simulink model "cordic_cycle"  (R2017a)
settings: Solver=FixedStepDiscrete  StartTime=0.0  StopTime=100  RelTol=1e-3  EnableMultiTasking=on
InitFcn:
  | %% DSPBuilder Start
  | alt_dspbuilder_update_model(bdroot)
  | %% DSPBuilder End
StartFcn:
  | %% DSPBuilder Start
  | alt_dspbuilder_hdlimport_prepare_for_simulation(bdroot)
  | %% DSPBuilder End
undefined symbols (not defined in the file or in its folder): AdvDSPBChannelOutDisplay, dpoly, dspba, dspba_ChannelInVis, dspba_ChannelOutVis, dspba_internal_get_channel_ports, evalAionMaskParam, latency, primtype, value
libraries: DSPBAPrim x101, DSPBAControl x12, DSPBABase x3, simulink x3
settings Model: Creator=lkong  LastModifiedBy=hatikvah
settings DataIOCC: LimitDataPoints=on  SaveFormat=Array  SignalLoggingSaveFormat=ModelDataLogs
settings OptimizationCC: ExpressionDepthLimit=2147483647  InitFltsAndDblsToZero=on  LifeSpan=inf
settings DebuggingCC: SaveWithParameterizedLinksMsg=none  UnderspecifiedInitializationDetection=Classic  MergeDetectMultiDrivingBlocksExec=none  SignalResolutionControl=TryResolveAllWithWarning  SolverPrmCheckMsg=warning  MultiTaskDSMMsg=warning  MultiTaskCondExecSysMsg=none  FcnCallInpInsideContextMsg=warning  StateNameClashWarn=warning  SFUnexpectedBacktrackingDiag=warning  SFNoUnconditionalDefaultTransitionDiag=warning  SFExecutionAtInitializationDiag=none
settings HardwareCC: ProdBitPerPointer=32  ProdBitPerSizeT=32  ProdBitPerPtrDiffT=32  ProdLargestAtomicFloat=None  ProdIntDivRoundTo=Undefined  ProdEndianess=Unspecified  ProdWordSize=32  ProdHWDeviceType=32-bit Generic
settings ModelReferenceCC: PropagateSignalLabelsOutOfModel=off
settings GRTTargetCC: TargetFcnLib=ansi_tfl_tmw.mat  TargetLangStandard=C89/C90 (ANSI)  GeneratePreprocessorConditionals=Disable all  CombineOutputUpdateFcns=off  GRTInterface=on
settings ConfigComp: CovMetricSettings=dw  CovHtmlReporting=on  CovSaveCumulativeToWorkspaceVar=on  CovSaveSingleToWorkspaceVar=on  CovExternalEMLEnable=off

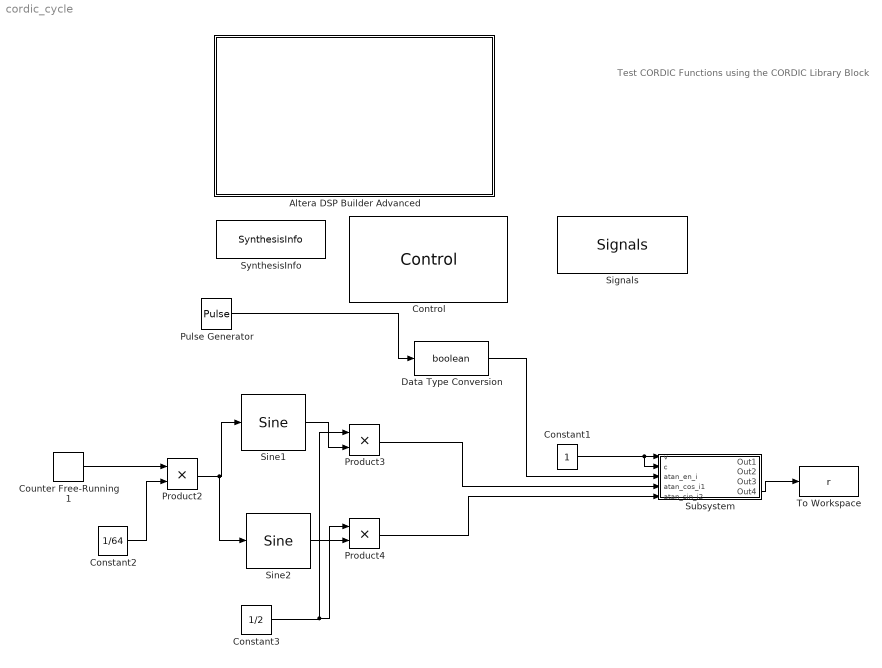
== system cordic_cycle ==
  note: Test CORDIC Functions
      | using the CORDIC Library Block
  Altera DSP Builder Advanced : Subsystem  mask(DSP Builder Advanced Blockset Ignored Block){}
      settings: OpenFcn=web('http://www.altera.com', '-new');
      mask Display: image(imread('intellogo.tif'));
  Constant1 : Constant  OutDataTypeStr=boolean  LockScale=on
  Constant2 : Constant  Value=1/64  OutDataTypeStr=double  LockScale=on
  Constant3 : Constant  Value=1/2  OutDataTypeStr=fixdt(1,32,31)  LockScale=on
  Control : DSPBABase/Control  generate=on  language=VHDL  destination=../rtl  destination_gui=../rtl  make_full_path=off  path_is_relative=on  autotestbench=on  signaldepth=3  coveragetestbench=off  logs=off  spacewidth=2  spacenum=1  addrwidth=10  datawidth=16  dataendian=Big Endian  hierarchicalnames=on  ramThresholdBits=20  distRamThresholdBits=-1  mlabThresholdBits=-1  hardMultiplierThresholdLuts=-1  version=20090407  errorOnChanMismatch=1  errorOnGPIOMismatch=0  importModelsimResults=0  cycleAccurate=off  reinterpretCastMult=off  paramFile=cordic_cycle_params.xml
  Counter Free-Running1 : simulink/Sources/Counter Free-Running  NumBits=10  tsamp=-1
  Data Type Conversion : DataTypeConversion  OutDataTypeStr=boolean
  Product2 : Product
  Product3 : Product  OutDataTypeStr=Inherit: Same as first input  LockScale=on
  Product4 : Product  OutDataTypeStr=Inherit: Same as first input  LockScale=on
  Pulse Generator : DiscretePulseGenerator  PulseType=Time based  Period=10  PulseWidth=2
  Signals : DSPBABase/Signals  clk=clk  freq=50  margin=0  rst=areset  rstactive=High  bus=bus  enbusclock=off  busfreq=50  bussync=off  version=20090407
  Sine1 : simulink/Lookup Tables/Sine  Formula=cos(2*pi*u)  NumDataPoints=(2^5)+1  OutputWordLength=32  InternalRulePriority=Speed
      settings: SourceProductName=Simulink
  Sine2 : simulink/Lookup Tables/Sine  Formula=sin(2*pi*u)  NumDataPoints=(2^5)+1  OutputWordLength=32  InternalRulePriority=Speed
      settings: SourceProductName=Simulink
  Subsystem : Subsystem
  SynthesisInfo : DSPBAPrim/SynthesisInfo  primtype=synthinfo  nInputs=0  nOutputs=0  omode=Inherit via internal rule  otype=sfix(16)  scale=2^-15  rndmethod=Truncate  factor=1  satmethod=Symmetric  shift_vec=[0 1 2 -1]  value=99  inPortNames=[' '; ' ';]  outPortNames=[' ']  dspbaimage=dspba_prim_ctrl.jpg  text=fprintf('Style=%s', style);  style=Scheduled  visibilities=2^17+2^18+2^19+2^20  constraintInUse=off  constraintRelation=>  constraintLimit=2  bitAccurate=off  version=20150220
  To Workspace : ToWorkspace  VariableName=r  SaveFormat=Timeseries  SampleTime=-1
  wires:
  Constant2/1 -> Product2/2
  Product2/1 -> Sine2/1, Sine1/1
  Product3/1 -> Subsystem/4(atan_cos_i1)
  Product4/1 -> Subsystem/5(atan_sin_i2)
  Pulse Generator/1 -> Data Type Conversion/1
  Sine1/1 -> Product3/2
  Sine2/1 -> Product4/2
  Constant3/1 -> Product4/1, Product3/1
  Counter Free-Running1/1 -> Product2/1
  Data Type Conversion/1 -> Subsystem/3(atan_en_i)
  Constant1/1 -> Subsystem/2(c), Subsystem/1(v)
  Subsystem/4(Out4) -> To Workspace/1

== system cordic_cycle/Altera DSP Builder Advanced ==

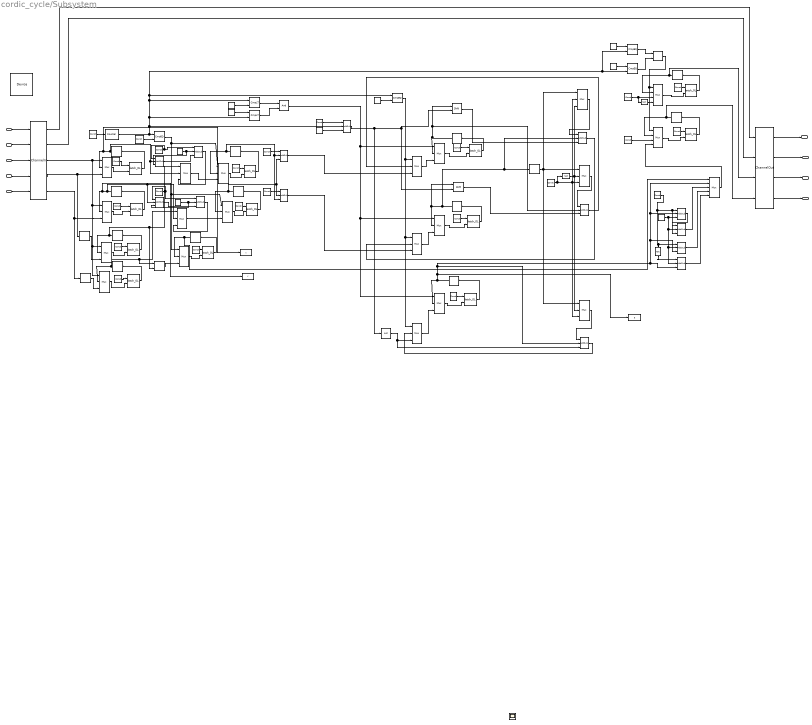
== system cordic_cycle/Subsystem ==
  v : Inport  OutDataTypeStr=boolean
  c : Inport  Port=2
  atan_en_i : Inport  Port=3
  atan_cos_i1 : Inport  Port=4
  atan_sin_i2 : Inport  Port=5
  AddSub{,1..13} (14 alike) : DSPBAPrim/AddSub  primtype=addsub  nInputs=3  nOutputs=1  omode=Inherit via internal rule  otype=sfix(16)  scale=2^-15  rndmethod=Unbiased  factor=1  satmethod=Symmetric  shift_vec=[0 1 2 -1]  value=0  inPortNames="['add'; 'x  '; 'y  ']"  outPortNames=[' ']  dspbaimage=dspba_prim.jpg  text=fprintf('add\nsub');  style=Optimised  visibilities=8+2^17+2^18  floatRounding=correct  advOptions=[]  version=20130110
  And : DSPBAPrim/And  primtype=and  nInputs=2  nOutputs=1  omode=Inherit via internal rule  otype=sfix(16)  scale=2^-15  rndmethod=Unbiased  factor=1  satmethod=Symmetric  shift_vec=[0 1 2 -1]  value=0  inPortNames=[' '; ' '; ' '; ' '; ' '; ' '; ' '; ' '; ' '; ' '; ' '; ' '; ' '; ' '; ' '; ' '; ]  outPortNames=[' ']  dspbaimage=dspba_prim.jpg  text=fprintf('&');  style=Optimised  visibilities=8+2  version=20090407
  BitCombine : DSPBAPrim/BitCombine  primtype=bitcombine  nInputs=2  nOutputs=1  omode=Inherit via internal rule  otype=sfix(16)  scale=2^-15  rndmethod=Unbiased  factor=1  satmethod=Symmetric  shift_vec=[0 1 2 -1]  value=0  inPortNames=['l'; 'h';]  outPortNames=[' ']  dspbaimage=dspba_prim.jpg  text=fprintf('[h,l]');  style=Optimised  visibilities=8+2  version=20090407
  BitCombine1 : DSPBAPrim/BitCombine  primtype=bitcombine  nInputs=2  nOutputs=1  omode=Inherit via internal rule  otype=sfix(16)  scale=2^-15  rndmethod=Unbiased  factor=1  satmethod=Symmetric  shift_vec=[0 1 2 -1]  value=0  inPortNames=['l'; 'h';]  outPortNames=[' ']  dspbaimage=dspba_prim.jpg  text=fprintf('[h,l]');  style=Optimised  visibilities=8+2  version=20090407
  ChannelIn : DSPBAPrim/ChannelIn  primtype=channelin  nInputs=dspba_internal_get_channel_ports(gcb)  nOutputs=dspba_internal_get_channel_ports(gcb)  omode=Inherit via internal rule  otype=sfix(16)  scale=2^-15  rndmethod=Unbiased  factor=1  satmethod=Symmetric  shift_vec=[0 1 2 -1]  value=3  inPortNames=['v'; 'c'; '0'; '1'; '2'; '3'; '4'; '5'; '6'; '7'; '8'; '9'; 'A'; 'B'; 'D'; 'E'; 'F'; 'G'; 'H'; 'I'; 'J'; 'K'; 'L'; 'M'; 'N'; 'O'; 'P'; 'Q'; 'R'; 'S'; 'T'; 'U'; 'W'; 'X'; 'Y'; 'Z']  outPortNames=['v'; 'c'; '0'; '1'; '2'; '3'; '4'; '5'; '6'; '7'; '8'; '9'; 'A'; 'B'; 'D'; 'E'; 'F'; 'G'; 'H'; 'I'; 'J'; 'K'; 'L'; 'M'; 'N'; 'O'; 'P'; 'Q'; 'R'; 'S'; 'T'; 'U'; 'W'; 'X'; 'Y'; 'Z']  dspbaimage=dspba_prim.jpg  text=fprintf('In');  style=Optimised  dataSignals=3  foldingEnabled=off  channels=1  sampleRate=200  packetBeginPresent=off  packetBeginEnabled=off  visibilities=dspba_ChannelInVis(gcb)  latencyCorrection=0  scheduleOrigin=off  version=20141013
  ChannelOut : DSPBAPrim/ChannelOut  primtype=channelout  nInputs=dspba_internal_get_channel_ports(gcb)  nOutputs=dspba_internal_get_channel_ports(gcb)  omode=Inherit via internal rule  otype=sfix(16)  scale=2^-15  rndmethod=Unbiased  factor=1  satmethod=Symmetric  shift_vec=[0 1 2 -1]  value=2  inPortNames=['v'; 'c'; '0'; '1'; '2'; '3'; '4'; '5'; '6'; '7'; '8'; '9'; 'A'; 'B'; 'D'; 'E'; 'F'; 'G'; 'H'; 'I'; 'J'; 'K'; 'L'; 'M'; 'N'; 'O'; 'P'; 'Q'; 'R'; 'S'; 'T'; 'U'; 'W'; 'X'; 'Y'; 'Z']  outPortNames=['v'; 'c'; '0'; '1'; '2'; '3'; '4'; '5'; '6'; '7'; '8'; '9'; 'A'; 'B'; 'D'; 'E'; 'F'; 'G'; 'H'; 'I'; 'J'; 'K'; 'L'; 'M'; 'N'; 'O'; 'P'; 'Q'; 'R'; 'S'; 'T'; 'U'; 'W'; 'X'; 'Y'; 'Z']  dspbaimage=dspba_prim.jpg  text=fprintf('Out%s', AdvDSPBChannelOutDisplay(latency));  style=Optimised  dataSignals=2  foldingEnabled=off  channels=1  sampleRate=200  packetBeginPresent=off  packetBeginEnabled=off  visibilities=dspba_ChannelOutVis(gcb)  latency=0  latencyCorrection=0  version=20141013
  ChooseBits : DSPBAPrim/ChooseBits  primtype=choosebits  nInputs=1  nOutputs=1  omode=Inherit via internal rule  otype=fixdt(0,1,1)  scale=1  rndmethod=Unbiased  factor=1  satmethod=Symmetric  shift_vec=[0 1 2 -1]  value=[31]  inPortNames=[' '; ' ';]  outPortNames=[' ']  dspbaimage=dspba_prim.jpg  text=fprintf('%s',dspba.perm2str(value));  style=Optimised  visibilities=1024  version=20090407
  ChooseBits1 : DSPBAPrim/ChooseBits  primtype=choosebits  nInputs=1  nOutputs=1  omode=Inherit via internal rule  otype=fixdt(0,1,1)  scale=1  rndmethod=Unbiased  factor=1  satmethod=Symmetric  shift_vec=[0 1 2 -1]  value=[31]  inPortNames=[' '; ' ';]  outPortNames=[' ']  dspbaimage=dspba_prim.jpg  text=fprintf('%s',dspba.perm2str(value));  style=Optimised  visibilities=1024  version=20090407
  ChooseBits2 : DSPBAPrim/ChooseBits  primtype=choosebits  nInputs=1  nOutputs=1  omode=Inherit via internal rule  otype=fixdt(0,1,1)  scale=1  rndmethod=Unbiased  factor=1  satmethod=Symmetric  shift_vec=[0 1 2 -1]  value=[31]  inPortNames=[' '; ' ';]  outPortNames=[' ']  dspbaimage=dspba_prim.jpg  text=fprintf('%s',dspba.perm2str(value));  style=Optimised  visibilities=1024  version=20090407
  CmpEQ{,1..3} (4 alike) : DSPBAPrim/CmpEQ  primtype=cmpeq  nInputs=2  nOutputs=1  omode=boolean  otype=sfix(16)  scale=2^-15  rndmethod=Unbiased  factor=1  satmethod=Symmetric  shift_vec=[0 1 2 -1]  value=0  inPortNames=[' '; ' ';]  outPortNames=[' ']  dspbaimage=dspba_prim.jpg  text=fprintf('==');  style=Optimised  visibilities=0  advOptions=[]  version=20130117
  CmpLT : DSPBAPrim/CmpLT  primtype=cmplt  nInputs=2  nOutputs=1  omode=boolean  otype=sfix(16)  scale=2^-15  rndmethod=Unbiased  factor=1  satmethod=Symmetric  shift_vec=[0 1 2 -1]  value=0  inPortNames=['a'; 'b';]  outPortNames=[' ']  dspbaimage=dspba_prim.jpg  text=fprintf('a<b');  style=Optimised  visibilities=0  advOptions=[]  version=20130117
  CmpLT1 : DSPBAPrim/CmpLT  primtype=cmplt  nInputs=2  nOutputs=1  omode=boolean  otype=sfix(16)  scale=2^-15  rndmethod=Unbiased  factor=1  satmethod=Symmetric  shift_vec=[0 1 2 -1]  value=0  inPortNames=['a'; 'b';]  outPortNames=[' ']  dspbaimage=dspba_prim.jpg  text=fprintf('a<b');  style=Optimised  visibilities=0  advOptions=[]  version=20130117
  Const{,2..4,6..7,10,15..16,22,24,28} (12 alike) : DSPBAPrim/Const  primtype=const  nInputs=0  nOutputs=1  omode=boolean  otype=sfix(32)  scale=2^-30  rndmethod=Unbiased  factor=1  satmethod=Symmetric  shift_vec=[0 1 2 -1]  value=1  inPortNames=['+'; '+';]  outPortNames=[' ']  dspbaimage=dspba_prim.jpg  text=fprintf('%s', num2str(value));  style=Optimised  visibilities=8 + 1024  floatPrecision=float32_m23  version=20120820
  Const1 : DSPBAPrim/Const  primtype=const  nInputs=0  nOutputs=1  omode=boolean  otype=sfix(16)  scale=2^-15  rndmethod=Unbiased  factor=1  satmethod=Symmetric  shift_vec=[0 1 2 -1]  value=1  inPortNames=['+'; '+';]  outPortNames=[' ']  dspbaimage=dspba_prim.jpg  text=fprintf('%s', num2str(value));  style=Optimised  visibilities=8 + 1024  floatPrecision=float32_m23  version=20120820
  Const11 : DSPBAPrim/Const  primtype=const  nInputs=0  nOutputs=1  omode=Specify via dialog  otype=sfix(32)  scale=2^-31  rndmethod=Unbiased  factor=1  satmethod=Symmetric  shift_vec=[0 1 2 -1]  value=-1  inPortNames=['+'; '+';]  outPortNames=[' ']  dspbaimage=dspba_prim.jpg  text=fprintf('%s', num2str(value));  style=Optimised  visibilities=8 + 1024  floatPrecision=float32_m23  version=20120820
  Const{9,12,19,21,25,27,31} (7 alike) : DSPBAPrim/Const  primtype=const  nInputs=0  nOutputs=1  omode=boolean  otype=sfix(16)  scale=2^-15  rndmethod=Unbiased  factor=1  satmethod=Symmetric  shift_vec=[0 1 2 -1]  value=0  inPortNames=['+'; '+';]  outPortNames=[' ']  dspbaimage=dspba_prim.jpg  text=fprintf('%s', num2str(value));  style=Optimised  visibilities=8 + 1024  floatPrecision=float32_m23  version=20120820
  Const13 : DSPBAPrim/Const  primtype=const  nInputs=0  nOutputs=1  omode=Specify via dialog  otype=ufix(6)  scale=2^0  rndmethod=Unbiased  factor=1  satmethod=Symmetric  shift_vec=[0 1 2 -1]  value=2  inPortNames=['+'; '+';]  outPortNames=[' ']  dspbaimage=dspba_prim.jpg  text=fprintf('%s', num2str(value));  style=Optimised  visibilities=8 + 1024  floatPrecision=float32_m23  version=20120820
  Const14 : DSPBAPrim/Const  primtype=const  nInputs=0  nOutputs=1  omode=Specify via dialog  otype=ufix(6)  scale=2^0  rndmethod=Unbiased  factor=1  satmethod=Symmetric  shift_vec=[0 1 2 -1]  value=34  inPortNames=['+'; '+';]  outPortNames=[' ']  dspbaimage=dspba_prim.jpg  text=fprintf('%s', num2str(value));  style=Optimised  visibilities=8 + 1024  floatPrecision=float32_m23  version=20120820
  Const17 : DSPBAPrim/Const  primtype=const  nInputs=0  nOutputs=1  omode=Specify via dialog  otype=ufix(6)  scale=2^0  rndmethod=Unbiased  factor=1  satmethod=Symmetric  shift_vec=[0 1 2 -1]  value=3  inPortNames=['+'; '+';]  outPortNames=[' ']  dspbaimage=dspba_prim.jpg  text=fprintf('%s', num2str(value));  style=Optimised  visibilities=8 + 1024  floatPrecision=float32_m23  version=20120820
  Const18 : DSPBAPrim/Const  primtype=const  nInputs=0  nOutputs=1  omode=boolean  otype=sfix(16)  scale=2^-15  rndmethod=Unbiased  factor=1  satmethod=Symmetric  shift_vec=[0 1 2 -1]  value=1  inPortNames=['+'; '+';]  outPortNames=[' ']  dspbaimage=dspba_prim.jpg  text=fprintf('%s', num2str(value));  style=Optimised  visibilities=8 + 1024  floatPrecision=float32_m23  version=20120820
  Const20 : DSPBAPrim/Const  primtype=const  nInputs=0  nOutputs=1  omode=Specify via dialog  otype=ufix(6)  scale=2^0  rndmethod=Unbiased  factor=1  satmethod=Symmetric  shift_vec=[0 1 2 -1]  value=3  inPortNames=['+'; '+';]  outPortNames=[' ']  dspbaimage=dspba_prim.jpg  text=fprintf('%s', num2str(value));  style=Optimised  visibilities=8 + 1024  floatPrecision=float32_m23  version=20120820
  Const23 : DSPBAPrim/Const  primtype=const  nInputs=0  nOutputs=1  omode=Specify via dialog  otype=ufix(6)  scale=2^0  rndmethod=Unbiased  factor=1  satmethod=Symmetric  shift_vec=[0 1 2 -1]  value=34  inPortNames=['+'; '+';]  outPortNames=[' ']  dspbaimage=dspba_prim.jpg  text=fprintf('%s', num2str(value));  style=Optimised  visibilities=8 + 1024  floatPrecision=float32_m23  version=20120820
  Const26 : DSPBAPrim/Const  primtype=const  nInputs=0  nOutputs=1  omode=Specify via dialog  otype=ufix(6)  scale=2^0  rndmethod=Unbiased  factor=1  satmethod=Symmetric  shift_vec=[0 1 2 -1]  value=35  inPortNames=['+'; '+';]  outPortNames=[' ']  dspbaimage=dspba_prim.jpg  text=fprintf('%s', num2str(value));  style=Optimised  visibilities=8 + 1024  floatPrecision=float32_m23  version=20120820
  Const29 : DSPBAPrim/Const  primtype=const  nInputs=0  nOutputs=1  omode=Specify via dialog  otype=sfix(32)  scale=2^-31  rndmethod=Unbiased  factor=1  satmethod=Symmetric  shift_vec=[0 1 2 -1]  value=0  inPortNames=['+'; '+';]  outPortNames=[' ']  dspbaimage=dspba_prim.jpg  text=fprintf('%s', num2str(value));  style=Optimised  visibilities=8 + 1024  floatPrecision=float32_m23  version=20120820
  Const30 : DSPBAPrim/Const  primtype=const  nInputs=0  nOutputs=1  omode=Specify via dialog  otype=sfix(32)  scale=2^-31  rndmethod=Unbiased  factor=1  satmethod=Symmetric  shift_vec=[0 1 2 -1]  value=-1  inPortNames=['+'; '+';]  outPortNames=[' ']  dspbaimage=dspba_prim.jpg  text=fprintf('%s', num2str(value));  style=Optimised  visibilities=8 + 1024  floatPrecision=float32_m23  version=20120820
  Const5 : DSPBAPrim/Const  primtype=const  nInputs=0  nOutputs=1  omode=Specify via dialog  otype=ufix(6)  scale=2^0  rndmethod=Unbiased  factor=1  satmethod=Symmetric  shift_vec=[0 1 2 -1]  value=2  inPortNames=['+'; '+';]  outPortNames=[' ']  dspbaimage=dspba_prim.jpg  text=fprintf('%s', num2str(value));  style=Optimised  visibilities=8 + 1024  floatPrecision=float32_m23  version=20120820
  Const8 : DSPBAPrim/Const  primtype=const  nInputs=0  nOutputs=1  omode=Specify via dialog  otype=sfix(32)  scale=2^-31  rndmethod=Unbiased  factor=1  satmethod=Symmetric  shift_vec=[0 1 2 -1]  value=-1  inPortNames=['+'; '+';]  outPortNames=[' ']  dspbaimage=dspba_prim.jpg  text=fprintf('%s', num2str(value));  style=Optimised  visibilities=8 + 1024  floatPrecision=float32_m23  version=20120820
  Counter : DSPBAPrim/Counter  primtype=counter  nInputs=1  nOutputs=1  omode=Inherit via internal rule  otype=uint(7)  scale=2^0  rndmethod=Unbiased  factor=1  satmethod=Symmetric  shift_vec=[0 1 2 -1]  value=[0 50 1]  inPortNames=[' '; ' ';]  outPortNames=[' ']  dspbaimage=dspba_prim.jpg  text=fprintf('counter\n[%d %d %d]', value(1), value(2), value(3));  style=Optimised  visibilities=8 + 1024  version=20090407
  Device : DSPBABase/Device  family=Arria 10  stratix4device=Stratix IV E  hardcopy4device=HardCopy IV E  stratix5device=Stratix V GX  device=AUTO  speed=1  stratixSpeed=-5  stratix2Speed=-3  stratix3Speed=-2  stratix4gxSpeed=-2  stratix4gtSpeed=-1  cyclone2Speed=-6  cyclone3Speed=-7  arria2Speed=-4  cyclone4eSpeed=-8  stratix5Speed=-3  arria5Speed=-4  arriaSpeed=-6  cyclone3lsSpeed=-7  cyclone5Speed=-6  arria2gzSpeed=-3  nightFurySpeed=-2  ecp2Speed=-7  hardcopycompat=off  version=20140217  max10flashmode=off  max10nomeminit=off
  Lut : DSPBAPrim/Lut  primtype=lut  nInputs=1  nOutputs=1  omode=Inherit via internal rule  otype=sfix(16)  scale=2^-15  rndmethod=Unbiased  factor=1  satmethod=Symmetric  shift_vec=[0 1 2 -1]  value=fi(atan(2.^(-1*(0:30))),1,32,31)./pi  inPortNames=[' '; ' ';]  outPortNames=[' ']  dspbaimage=dspba_prim.jpg  text=fprintf('LUT');  style=Optimised  visibilities=8 + 1024  floatPrecision=float32_m23  version=20090407
  Mux{,1..17} (18 alike) : DSPBAPrim/Mux  primtype=mux  nInputs=evalAionMaskParam(gcb,'value',1)+1  nOutputs=1  omode=Inherit via internal rule  otype=sfix(16)  scale=2^-15  rndmethod=Unbiased  factor=1  satmethod=Symmetric  shift_vec=[0 1 2 -1]  value=2  inPortNames=['s '; 'd0'; 'd1'; 'd2'; 'd3'; 'd4'; 'd5'; 'd6'; 'd7'; 'd8'; 'd9';]  outPortNames=[' ']  dspbaimage=dspba_prim.jpg  text=fprintf('%s', primtype);  style=Optimised  visibilities=1032  version=20131025
  Mux18 : DSPBAPrim/Mux  primtype=mux  nInputs=evalAionMaskParam(gcb,'value',1)+1  nOutputs=1  omode=Inherit via internal rule  otype=sfix(16)  scale=2^-15  rndmethod=Unbiased  factor=1  satmethod=Symmetric  shift_vec=[0 1 2 -1]  value=4  inPortNames=['s '; 'd0'; 'd1'; 'd2'; 'd3'; 'd4'; 'd5'; 'd6'; 'd7'; 'd8'; 'd9';]  outPortNames=[' ']  dspbaimage=dspba_prim.jpg  text=fprintf('%s', primtype);  style=Optimised  visibilities=1032  version=20131025
  Mux19 : DSPBAPrim/Mux  primtype=mux  nInputs=evalAionMaskParam(gcb,'value',1)+1  nOutputs=1  omode=Inherit via internal rule  otype=sfix(16)  scale=2^-15  rndmethod=Unbiased  factor=1  satmethod=Symmetric  shift_vec=[0 1 2 -1]  value=3  inPortNames=['s '; 'd0'; 'd1'; 'd2'; 'd3'; 'd4'; 'd5'; 'd6'; 'd7'; 'd8'; 'd9';]  outPortNames=[' ']  dspbaimage=dspba_prim.jpg  text=fprintf('%s', primtype);  style=Optimised  visibilities=1032  version=20131025
  Mux20 : DSPBAPrim/Mux  primtype=mux  nInputs=evalAionMaskParam(gcb,'value',1)+1  nOutputs=1  omode=Inherit via internal rule  otype=sfix(16)  scale=2^-15  rndmethod=Unbiased  factor=1  satmethod=Symmetric  shift_vec=[0 1 2 -1]  value=3  inPortNames=['s '; 'd0'; 'd1'; 'd2'; 'd3'; 'd4'; 'd5'; 'd6'; 'd7'; 'd8'; 'd9';]  outPortNames=[' ']  dspbaimage=dspba_prim.jpg  text=fprintf('%s', primtype);  style=Optimised  visibilities=1032  version=20131025
  Not : DSPBAPrim/Not  primtype=not  nInputs=1  nOutputs=1  omode=Inherit via internal rule  otype=sfix(16)  scale=2^-15  rndmethod=Unbiased  factor=1  satmethod=Symmetric  shift_vec=[0 1 2 -1]  value=0  inPortNames=[' '; ' ';]  outPortNames=[' ']  dspbaimage=dspba_prim.jpg  text=fprintf('~');  style=Optimised  visibilities=8  version=20090407
  Not1 : DSPBAPrim/Not  primtype=not  nInputs=1  nOutputs=1  omode=Inherit via internal rule  otype=sfix(16)  scale=2^-15  rndmethod=Unbiased  factor=1  satmethod=Symmetric  shift_vec=[0 1 2 -1]  value=0  inPortNames=[' '; ' ';]  outPortNames=[' ']  dspbaimage=dspba_prim.jpg  text=fprintf('~');  style=Optimised  visibilities=8  version=20090407
  Not2 : DSPBAPrim/Not  primtype=not  nInputs=1  nOutputs=1  omode=Inherit via internal rule  otype=sfix(16)  scale=2^-15  rndmethod=Unbiased  factor=1  satmethod=Symmetric  shift_vec=[0 1 2 -1]  value=0  inPortNames=[' '; ' ';]  outPortNames=[' ']  dspbaimage=dspba_prim.jpg  text=fprintf('~');  style=Optimised  visibilities=8  version=20090407
  SampleDelay{,1,5..9,11} (8 alike) : DSPBAPrim/SampleDelay  primtype=sampdelay  nInputs=1  nOutputs=1  omode=Specify via dialog  otype=sfix(32)  scale=2^-31  rndmethod=Unbiased  factor=1  satmethod=Symmetric  shift_vec=[0 1 2 -1]  value=1  inPortNames=[' '; ' ';]  outPortNames=[' ']  dspbaimage=dspba_prim.jpg  text=dpoly(1, eye(1,value+1), 'z')  style=Optimised  visibilities=8 + 1024  flexible=off  slackgroup=0  augmented=0  version=20090407  advOptions=[]
  SampleDelay10 : DSPBAPrim/SampleDelay  primtype=sampdelay  nInputs=1  nOutputs=1  omode=boolean  otype=sfix(32)  scale=2^-31  rndmethod=Unbiased  factor=1  satmethod=Symmetric  shift_vec=[0 1 2 -1]  value=1  inPortNames=[' '; ' ';]  outPortNames=[' ']  dspbaimage=dspba_prim.jpg  text=dpoly(1, eye(1,value+1), 'z')  style=Optimised  visibilities=8 + 1024  flexible=off  slackgroup=0  augmented=0  version=20090407  advOptions=[]
  SampleDelay2 : DSPBAPrim/SampleDelay  primtype=sampdelay  nInputs=1  nOutputs=1  omode=boolean  otype=sfix(32)  scale=2^-30  rndmethod=Unbiased  factor=1  satmethod=Symmetric  shift_vec=[0 1 2 -1]  value=1  inPortNames=[' '; ' ';]  outPortNames=[' ']  dspbaimage=dspba_prim.jpg  text=dpoly(1, eye(1,value+1), 'z')  style=Optimised  visibilities=8 + 1024  flexible=off  slackgroup=0  augmented=0  version=20090407  advOptions=[]
  SampleDelay3 : DSPBAPrim/SampleDelay  primtype=sampdelay  nInputs=1  nOutputs=1  omode=boolean  otype=sfix(32)  scale=2^-30  rndmethod=Unbiased  factor=1  satmethod=Symmetric  shift_vec=[0 1 2 -1]  value=1  inPortNames=[' '; ' ';]  outPortNames=[' ']  dspbaimage=dspba_prim.jpg  text=dpoly(1, eye(1,value+1), 'z')  style=Optimised  visibilities=8 + 1024  flexible=off  slackgroup=0  augmented=0  version=20090407  advOptions=[]
  SampleDelay4 : DSPBAPrim/SampleDelay  primtype=sampdelay  nInputs=1  nOutputs=1  omode=Specify via dialog  otype=ufix(2)  scale=2^0  rndmethod=Unbiased  factor=1  satmethod=Symmetric  shift_vec=[0 1 2 -1]  value=1  inPortNames=[' '; ' ';]  outPortNames=[' ']  dspbaimage=dspba_prim.jpg  text=dpoly(1, eye(1,value+1), 'z')  style=Optimised  visibilities=8 + 1024  flexible=off  slackgroup=0  augmented=0  version=20090407  advOptions=[]
  Scope : Scope
  Shift : DSPBAPrim/Shift  primtype=shift  nInputs=2  nOutputs=1  omode=Specify via dialog  otype=sfix(32)  scale=2^-31  rndmethod=Unbiased  factor=1  satmethod=Symmetric  shift_vec=[0 1 2 -1]  value=0  inPortNames=['a'; 'b';]  outPortNames=[' ']  dspbaimage=dspba_prim.jpg  text=fprintf('a >> b');  style=Optimised  visibilities=8  version=20090407
  Shift1 : DSPBAPrim/Shift  primtype=shift  nInputs=2  nOutputs=1  omode=Specify via dialog  otype=sfix(32)  scale=2^-31  rndmethod=Unbiased  factor=1  satmethod=Symmetric  shift_vec=[0 1 2 -1]  value=0  inPortNames=['a'; 'b';]  outPortNames=[' ']  dspbaimage=dspba_prim.jpg  text=fprintf('a >> b');  style=Optimised  visibilities=8  version=20090407
  To Workspace : ToWorkspace  VariableName=x  SaveFormat=Timeseries  SampleTime=-1
  To Workspace1 : ToWorkspace  VariableName=y  SaveFormat=Timeseries  SampleTime=-1
  To Workspace2 : ToWorkspace  VariableName=a  SaveFormat=Timeseries  SampleTime=-1
  s_a_ok : DSPBAControl/latch_0L
  s_a_res : DSPBAControl/latch_0L
  s_ang : DSPBAControl/latch_0L
  "s_quadrant " : DSPBAControl/latch_0L
  s_x : DSPBAControl/latch_0L
  s_x_0 : DSPBAControl/latch_0L
  s_x_1 : DSPBAControl/latch_0L
  s_x_is_n : DSPBAControl/latch_0L
  s_y : DSPBAControl/latch_0L
  s_y_0 : DSPBAControl/latch_0L
  s_y_1 : DSPBAControl/latch_0L
  s_y_is_n1 : DSPBAControl/latch_0L
  Out1 : Outport
  Out2 : Outport  Port=2
  Out3 : Outport  Port=3
  Out4 : Outport  Port=4
  wires:
  ChannelIn/4 -> Mux/3, ChooseBits/1
  s_x_0/1 -> SampleDelay/1
  ChannelIn/5 -> ChooseBits1/1, Mux1/3
  Mux1/1 -> s_y_0/2
  Const1/1 -> s_y_0/1
  s_y_0/1 -> SampleDelay1/1
  SampleDelay/1 -> Mux8/2, AddSub3/2, To Workspace/1, Mux/2
  SampleDelay1/1 -> AddSub1/2, Mux6/2, To Workspace1/1, Mux1/2
  Const/1 -> s_x_0/1
  Mux/1 -> s_x_0/2
  ChannelIn/3 -> Mux3/1, Mux2/1, Mux1/1, Mux/1
  Const2/1 -> Counter/1
  Const3/1 -> s_x_is_n/1
  SampleDelay2/1 -> Mux8/1, BitCombine/2, Mux2/2
  s_x_is_n/1 -> SampleDelay2/1
  Mux2/1 -> s_x_is_n/2
  ChooseBits/1 -> Mux2/3
  s_y_is_n1/1 -> SampleDelay3/1
  Const4/1 -> s_y_is_n1/1
  Mux3/1 -> s_y_is_n1/2
  SampleDelay3/1 -> Mux3/2, Mux6/1, BitCombine/1
  ChooseBits1/1 -> Mux3/3
  Counter/1 -> CmpEQ3/2, CmpEQ2/2, CmpEQ1/1, CmpLT1/1, CmpLT/2, AddSub6/2, CmpEQ/1
  Const5/1 -> CmpEQ/2
  CmpEQ/1 -> Mux4/1, Mux5/1, Mux7/1
  BitCombine/1 -> Mux4/3
  Const6/1 -> "s_quadrant "/1
  Mux4/1 -> "s_quadrant "/2
  "s_quadrant "/1 -> SampleDelay4/1
  Const7/1 -> s_y_1/1
  s_y_1/1 -> SampleDelay5/1
  SampleDelay5/1 -> AddSub5/2, AddSub4/3, Mux5/2
  Mux5/1 -> s_y_1/2
  Mux6/1 -> Mux5/3
  Const9/1 -> AddSub/1, AddSub1/1
  Const8/1 -> AddSub/2, AddSub1/3
  AddSub1/1 -> AddSub/3
  AddSub/1 -> Mux6/3
  Const10/1 -> s_x_1/1
  Mux7/1 -> s_x_1/2
  s_x_1/1 -> SampleDelay6/1
  SampleDelay6/1 -> AddSub5/3, AddSub4/2, Mux7/2
  Mux8/1 -> Mux7/3
  Const11/1 -> AddSub3/3, AddSub2/2
  Const12/1 -> AddSub2/1, AddSub3/1
  AddSub3/1 -> AddSub2/3
  AddSub2/1 -> Mux8/3
  Const13/1 -> CmpLT/1
  Const14/1 -> CmpLT1/2
  CmpLT1/1 -> And/1
  CmpLT/1 -> And/2
  Const15/1 -> s_x/1
  s_x/1 -> SampleDelay7/1
  SampleDelay7/1 -> AddSub8/2, Shift/1, Mux9/2
  Mux9/1 -> s_x/2
  And/1 -> Mux15/1, Mux10/1, Mux9/1
  Const16/1 -> s_y/1
  Mux10/1 -> s_y/2
  s_y/1 -> SampleDelay8/1
  SampleDelay8/1 -> AddSub9/2, ChooseBits2/1, Shift1/1, Mux10/2
  Const17/1 -> CmpEQ1/2
  CmpEQ1/1 -> Mux16/1, Mux12/1, Mux11/1
  Const18/1 -> AddSub4/1
  Const19/1 -> AddSub5/1
  AddSub4/1 -> Mux11/3
  AddSub5/1 -> Mux12/3
  Mux11/1 -> Mux9/3
  Mux12/1 -> Mux10/3
  Const20/1 -> AddSub6/3
  Const21/1 -> AddSub6/1
  Shift1/1 -> AddSub8/3
  Const25/1 -> Not/1, Mux17/3, Mux14/2, Mux13/3
  Not/1 -> Mux14/3, Mux17/2, Mux13/2
  Mux13/1 -> AddSub8/1
  AddSub8/1 -> Mux11/2
  Mux14/1 -> AddSub9/1
  Shift/1 -> AddSub9/3
  AddSub9/1 -> Mux12/2
  Const22/1 -> s_ang/1
  s_ang/1 -> SampleDelay9/1
  Mux15/1 -> s_ang/2
  Mux16/1 -> Mux15/3
  ChooseBits2/1 -> Mux14/1, Mux13/1, Mux17/1
  Mux17/1 -> AddSub7/1
  AddSub7/1 -> Mux16/2
  AddSub6/1 -> Lut/1, Shift/2, Shift1/2
  Lut/1 -> AddSub7/3, Mux16/3
  Const23/1 -> CmpEQ2/1
  Const24/1 -> s_a_ok/1
  Mux19/1 -> s_a_ok/2
  s_a_ok/1 -> SampleDelay10/1
  SampleDelay10/1 -> Mux19/2, ChannelOut/3
  Const26/1 -> CmpEQ3/1
  CmpEQ2/1 -> BitCombine1/2
  CmpEQ3/1 -> BitCombine1/1
  BitCombine1/1 -> Mux20/1, Mux19/1
  Const27/1 -> Not1/1, Mux19/3
  Not1/1 -> Mux19/4
  Const28/1 -> s_a_res/1
  Mux20/1 -> s_a_res/2
  s_a_res/1 -> SampleDelay11/1
  SampleDelay11/1 -> ChannelOut/4, Mux20/2
  Const29/1 -> Mux20/3
  Mux18/1 -> Mux20/4
  Const31/1 -> Not2/1, AddSub12/1, AddSub11/1, AddSub10/1
  Const30/1 -> AddSub13/2, AddSub12/2, AddSub11/2, AddSub10/3
  AddSub10/1 -> AddSub11/3
  AddSub11/1 -> Mux18/3
  Not2/1 -> AddSub13/1
  AddSub12/1 -> Mux18/4
  AddSub13/1 -> Mux18/5
  SampleDelay9/1 -> To Workspace2/1, AddSub13/3, AddSub12/3, AddSub10/2, Mux18/2, AddSub7/2, Mux15/2
  SampleDelay4/1 -> Mux18/1, Mux4/2
  ChannelIn/1 -> ChannelOut/1
  ChannelIn/2 -> ChannelOut/2
  v/1 -> ChannelIn/1
  c/1 -> ChannelIn/2
  atan_en_i/1 -> ChannelIn/3
  atan_cos_i1/1 -> ChannelIn/4
  atan_sin_i2/1 -> ChannelIn/5
  ChannelOut/1 -> Out1/1
  ChannelOut/2 -> Out2/1
  ChannelOut/3 -> Out3/1
  ChannelOut/4 -> Out4/1
